simulink model "System"  (R2016b)
settings: Solver=ode45  StartTime=0.0  StopTime=simulatietijd  RelTol=1e-3  EnableMultiTasking=on
values from neighbouring files (symbols this model uses):
  beta = toeplitz(C,R)    [Torricelli_DMC_uitvoeren.m]    (also in optimisation.m; parameter_optimalisatie.m; script.m; variatie_m.m)
  h0 = 0    [Torricelli_DMC_uitvoeren.m]    (also in optimisation.m; parameter_optimalisatie.m; script.m; variatie_m.m)
  hna = 8    [Torricelli_DMC_uitvoeren.m]    (also in optimisation.m; parameter_optimalisatie.m; script.m; variatie_m.m)
  hvoor = 3    [Torricelli_DMC_uitvoeren.m]    (also in optimisation.m; parameter_optimalisatie.m; script.m; variatie_m.m)
  K = 0.3    [Torricelli_DMC_uitvoeren.m]    (also in optimisation.m = K_help(j); parameter_optimalisatie.m = K_good; script.m; variatie_m.m)
  staptijd = 1000    [Torricelli_DMC_uitvoeren.m]    (also in optimisation.m; parameter_optimalisatie.m; script.m; variatie_m.m)
  Ts = round(1/7.5*tau)    [Torricelli_DMC_uitvoeren.m]    (also in optimisation.m; parameter_optimalisatie.m; script.m; variatie_m.m)
  u0 = 0    [Torricelli_DMC_uitvoeren.m]    (also in discrete_DMC.m; optimisation.m; parameter_optimalisatie.m; script.m)
settings Model: Creator=Tim  LastModifiedBy=wrquaghe
settings DataIOCC: LimitDataPoints=on  SaveFormat=Array
settings OptimizationCC: LifeSpan=inf
settings DebuggingCC: AllowSymbolicDim=off  SFUnexpectedBacktrackingDiag=warning  SFNoUnconditionalDefaultTransitionDiag=warning  SFExecutionAtInitializationDiag=none
settings HardwareCC: ProdBitPerPointer=32  ProdBitPerSizeT=32  ProdBitPerPtrDiffT=32  ProdLargestAtomicFloat=None  ProdIntDivRoundTo=Undefined  ProdEndianess=Unspecified  ProdWordSize=32  ProdHWDeviceType=32-bit Generic
settings ModelReferenceCC: PropagateSignalLabelsOutOfModel=off
settings GRTTargetCC: TargetLangStandard=C89/C90 (ANSI)  GeneratePreprocessorConditionals=Disable all
settings ConfigComp: CovMetricSettings=dw  CovHtmlReporting=on  CovSaveCumulativeToWorkspaceVar=on  CovSaveSingleToWorkspaceVar=on  CovExternalEMLEnable=off

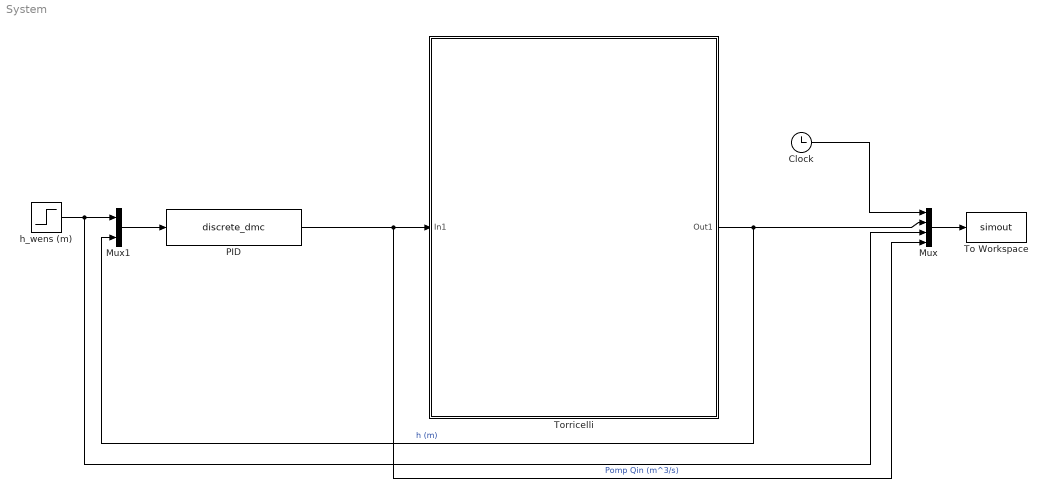
== system System ==
  Clock : Clock
  Mux : Mux
  Mux1 : Mux  Inputs=2
  PID : S-Function  FunctionName=discrete_dmc  Parameters=beta,K,Ts,u0  SFunctionDeploymentMode=off  EnableBusSupport=off
  To Workspace : ToWorkspace  VariableName=simout  SampleTime=-1
  Torricelli : Subsystem
      mask Display: image(imread('torricelli.png'))
  h_wens (m) : Step  Time=staptijd  Before=hvoor  After=hna  SampleTime=0
  wires:
  Mux/1 -> To Workspace/1
  Clock/1 -> Mux/1
  Torricelli/1(Out1) -> Mux1/2, Mux/2  "h (m)"
  h_wens (m)/1 -> Mux/3, Mux1/1
  Mux1/1 -> PID/1
  PID/1 -> Mux/4, Torricelli/1(In1)  "Pomp Qin (m^3/s)"

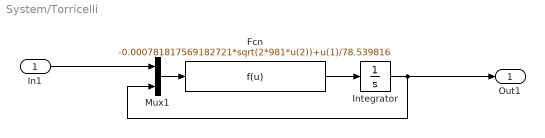
== system System/Torricelli ==
  In1 : Inport
  Fcn : Fcn  Expr=-0.000781817569182721*sqrt(2*981*u(2))+u(1)/78.539816
  Integrator : Integrator  InitialCondition=h0
  Mux1 : Mux  Inputs=2
  Out1 : Outport
  wires:
  Integrator/1 -> Mux1/2, Out1/1
  Mux1/1 -> Fcn/1
  Fcn/1 -> Integrator/1
  In1/1 -> Mux1/1
